simulink model "simulink1"  (R2018b)
settings: Solver=VariableStepAuto  StartTime=0.0  StopTime=10.0  RelTol=1e-3
libraries: simulink x3
settings Model: Creator=DEMİREL  LastModifiedBy=DEMİREL

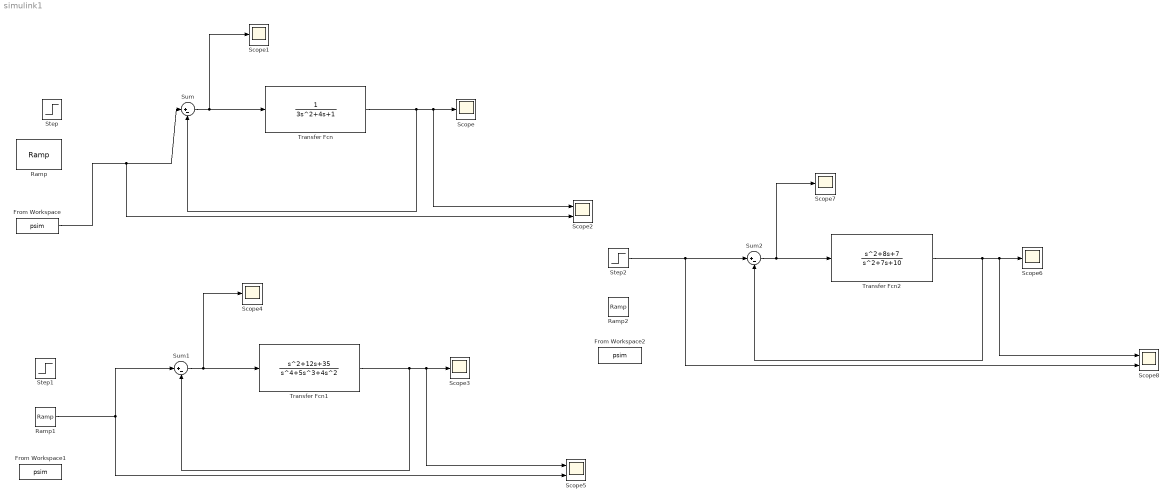
== system simulink1 ==
  From Workspace : FromWorkspace  VariableName=psim  SampleTime=0
  From Workspace1 : FromWorkspace  VariableName=psim  SampleTime=0
  From Workspace2 : FromWorkspace  VariableName=psim  SampleTime=0
  Ramp : simulink/Sources/Ramp  slope=1  start=0  InitialOutput=0
  Ramp1 : simulink/Sources/Ramp  slope=1  start=0  InitialOutput=0
  Ramp2 : simulink/Sources/Ramp  slope=1  start=0  InitialOutput=0
  Scope{,1,3..4,6..7} (6 alike) : Scope
  Scope2 : Scope  NumInputPorts=2
  Scope5 : Scope  NumInputPorts=2
  Scope8 : Scope  NumInputPorts=2
  Step : Step  SampleTime=0
  Step1 : Step  SampleTime=0
  Step2 : Step  SampleTime=0
  Sum : Sum  Inputs=|+-
  Sum1 : Sum  Inputs=|+-
  Sum2 : Sum  Inputs=|+-
  Transfer Fcn : TransferFcn  Denominator=[3 4 1]
  Transfer Fcn1 : TransferFcn  Numerator=[1 12 35]  Denominator=[1 5 4 0 0 ]
  Transfer Fcn2 : TransferFcn  Numerator=[1 8 7]  Denominator=[1 7 10]
  wires:
  Sum/1 -> Scope1/1, Transfer Fcn/1
  Transfer Fcn/1 -> Sum/2, Scope2/1, Scope/1
  Sum1/1 -> Scope4/1, Transfer Fcn1/1
  Transfer Fcn1/1 -> Sum1/2, Scope5/1, Scope3/1
  Sum2/1 -> Scope7/1, Transfer Fcn2/1
  Transfer Fcn2/1 -> Sum2/2, Scope8/1, Scope6/1
  Step2/1 -> Scope8/2, Sum2/1
  Ramp1/1 -> Sum1/1, Scope5/2
  From Workspace/1 -> Scope2/2, Sum/1
